simulink model "AMCLIB_SpeedLoop_BAM_FLT"  (Simulink 8.3)
settings: Solver=ode45  StartTime=0.0  StopTime=10.0  RelTol=1e-3
undefined symbols (not defined in the file): fltIntegGainQ, fltLambdaW, fltPropGainQ, fltRampDown, fltRampUp
settings Model: Creator=B37097  LastModifiedBy=B37097
settings DataIOCC: SignalLoggingSaveFormat=Dataset
settings DebuggingCC: UnderspecifiedInitializationDetection=Simplified  StateNameClashWarn=none
settings GRTTargetCC: CombineOutputUpdateFcns=on  GRTInterface=off

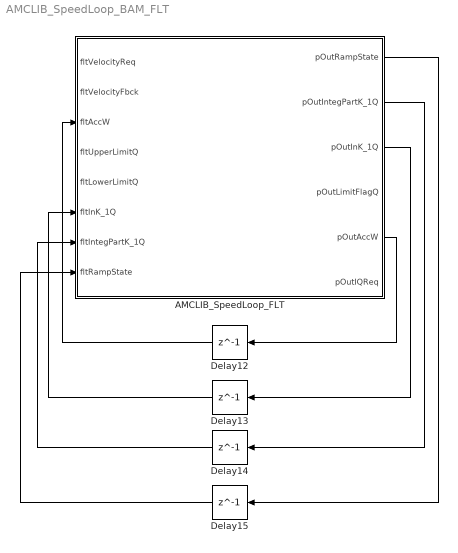
== system AMCLIB_SpeedLoop_BAM_FLT ==
  AMCLIB_SpeedLoop_FLT : Subsystem  mask(AMCLIB_SpeedLoop_FLT){fltLambdaW=fltLambdaW, fltPropGainQ=fltPropGainQ, fltIntegGainQ=fltIntegGainQ, fltRampUp=fltRampUp, fltRampDown=fltRampDown}
      mask help: Bit accurate model of the speed loop algorithm with field weakening capability. All parameters as well as input and output values are in single precision floating data format.
      mask init:
      | pos = get_param(gcb, 'Position');width = pos(3) - pos(1); height = pos(4) - pos(2);tX=width/2;tY=height*0.9;
      mask Display: color('black');port_label('input',1,'fltVelocityReq');port_label('input',2,'fltVelocityFbck');port_label('input',3,'fltAccW');port_label('input',4,'fltUpperLimitQ');port_label('input',5,'fltLowerLimitQ');port_label('input',6,'fltInK_1Q');port_label('input',7,'fltIntegPartK_1Q');port_label('input',8,'fltRampState');port_label('output',1,'pOutRampState');port_label('output',2,'pOutIntegPartK_1Q');port_label('output',3,'pOutInK_1Q');port_label('output',4,'pOutLimitFlagQ');port_label('output',5,'pOutAccW');port_label('output',6,'pOutIQReq');color('black');disp('AMCLIB_SpeedLoop_FLT');color('blue');text(tX,tY, 'BAM', 'horizontalAlignment', 'center');
  Delay{12..15} (4 alike) : Delay  DelayLength=1  InitialCondition=0
  wires:
  AMCLIB_SpeedLoop_FLT/5(pOutAccW) -> Delay12/1
  AMCLIB_SpeedLoop_FLT/3(pOutInK_1Q) -> Delay13/1
  AMCLIB_SpeedLoop_FLT/2(pOutIntegPartK_1Q) -> Delay14/1
  AMCLIB_SpeedLoop_FLT/1(pOutRampState) -> Delay15/1
  Delay12/1 -> AMCLIB_SpeedLoop_FLT/3(fltAccW)
  Delay13/1 -> AMCLIB_SpeedLoop_FLT/6(fltInK_1Q)
  Delay14/1 -> AMCLIB_SpeedLoop_FLT/7(fltIntegPartK_1Q)
  Delay15/1 -> AMCLIB_SpeedLoop_FLT/8(fltRampState)

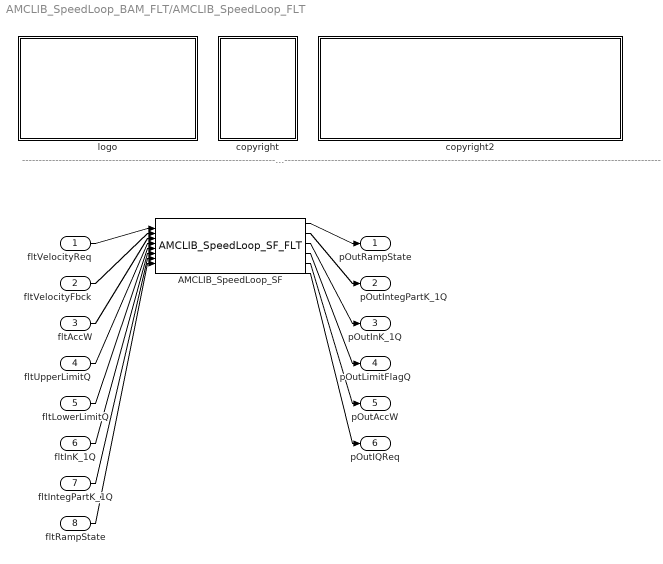
== system AMCLIB_SpeedLoop_BAM_FLT/AMCLIB_SpeedLoop_FLT ==
  note: ---------------------------------------------------------------------------------------------------------------------------------------------------------------------------------------------------
  fltVelocityReq : Inport
  fltVelocityFbck : Inport  Port=2
  fltAccW : Inport  Port=3
  fltUpperLimitQ : Inport  Port=4
  fltLowerLimitQ : Inport  Port=5
  fltInK_1Q : Inport  Port=6
  fltIntegPartK_1Q : Inport  Port=7
  fltRampState : Inport  Port=8
  AMCLIB_SpeedLoop_SF : S-Function  FunctionName=AMCLIB_SpeedLoop_SF_FLT  Parameters=fltLambdaW,fltPropGainQ,fltIntegGainQ,fltRampUp,fltRampDown  EnableBusSupport=off
  copyright : Subsystem
      mask Display: text(10,90,'FILE:');text(10,75,'DESRIPTION:');text(10,60,'COPYRIGHT:');text(10,45,'VERSION:');text(10,30,'DATE:')
  copyright2 : Subsystem
      mask Display: text(10,90,'AMCLIB_SpeedLoop_BAM_FLT.mdl');text(10,75,'Speed Loop with Field Weakening.');text(10,60,'NXP');text(10,45,'1.0');text(10,30,'28-Aug-2017');
  logo : Subsystem
      mask Display: image(imread('logo.jpg'))
  pOutRampState : Outport
  pOutIntegPartK_1Q : Outport  Port=2
  pOutInK_1Q : Outport  Port=3
  pOutLimitFlagQ : Outport  Port=4
  pOutAccW : Outport  Port=5
  pOutIQReq : Outport  Port=6
  wires:
  fltVelocityReq/1 -> AMCLIB_SpeedLoop_SF/1
  fltVelocityFbck/1 -> AMCLIB_SpeedLoop_SF/2
  fltAccW/1 -> AMCLIB_SpeedLoop_SF/3
  fltUpperLimitQ/1 -> AMCLIB_SpeedLoop_SF/4
  fltLowerLimitQ/1 -> AMCLIB_SpeedLoop_SF/5
  fltInK_1Q/1 -> AMCLIB_SpeedLoop_SF/6
  fltIntegPartK_1Q/1 -> AMCLIB_SpeedLoop_SF/7
  fltRampState/1 -> AMCLIB_SpeedLoop_SF/8
  AMCLIB_SpeedLoop_SF/1 -> pOutRampState/1
  AMCLIB_SpeedLoop_SF/2 -> pOutIntegPartK_1Q/1
  AMCLIB_SpeedLoop_SF/3 -> pOutInK_1Q/1
  AMCLIB_SpeedLoop_SF/4 -> pOutLimitFlagQ/1
  AMCLIB_SpeedLoop_SF/5 -> pOutAccW/1
  AMCLIB_SpeedLoop_SF/6 -> pOutIQReq/1

== system AMCLIB_SpeedLoop_BAM_FLT/AMCLIB_SpeedLoop_FLT/copyright ==

== system AMCLIB_SpeedLoop_BAM_FLT/AMCLIB_SpeedLoop_FLT/copyright2 ==

== system AMCLIB_SpeedLoop_BAM_FLT/AMCLIB_SpeedLoop_FLT/logo ==
